simulink model "power_switching"  (Simulink 6.0)
settings: Solver=ode15s  SolverMode=SingleTasking  StartTime=0.0  StopTime=.2  RelTol=1e-4
libraries: powerlib x12, powerlib_extras x1
settings Model: Creator=patrice  LastModifiedBy=batserve  ExtModeTrigMode=oneshot  ExtModeArmWhenConnect=off  ExtModeAutoUpdateStatusClock=off
settings DataIOCC: LimitDataPoints=off  SignalLoggingName=sigsOut
settings OptimizationCC: BlockReduction=off  BooleanDataType=off
settings DebuggingCC: CheckExecutionContextPreStartOutputMsg=on  CheckExecutionContextRuntimeOutputMsg=on  SolverPrmCheckMsg=none  UnconnectedInputMsg=none  UnconnectedOutputMsg=none
settings HardwareCC: TargetUnknown=on
settings RTWCC: TemplateMakefile=grt_vc.tmf

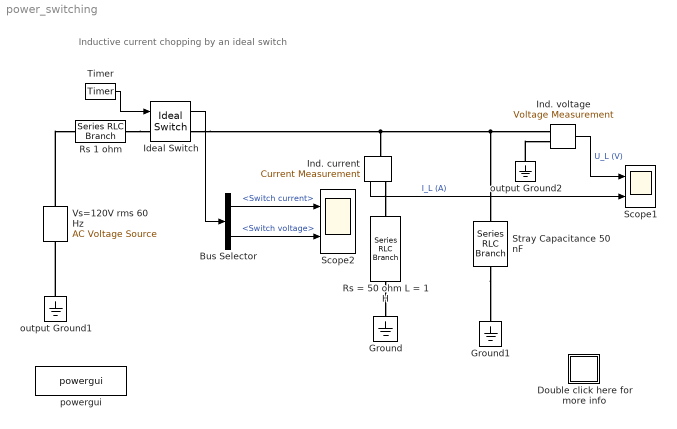
== system power_switching ==
  note: Inductive current chopping by an ideal switch
  "  Ind. current" : powerlib/Measurements/Current Measurement  Tag=PoWeRsYsTeMmEaSuReMeNt  Orientation=down  PhasorSimulation=off  OutputType=Magnitude  PSBequivalent=0
  Bus Selector : BusSelector  DialogController=Simulink.DDGSource_Bus  OutputSignals=Switch current,Switch voltage
  Double click here for more info : Subsystem
      mask Display: disp('?')
  Ground : powerlib/Elements/Ground  Orientation=down  PhysicalDomain=powersysdomain  SubClassName=unknown  LeftPortType=p1  RightPortType=p1  LConnTagsString=a
  Ground1 : powerlib/Elements/Ground  Orientation=down  PhysicalDomain=powersysdomain  SubClassName=unknown  LeftPortType=p1  RightPortType=p1  LConnTagsString=a
  Ideal Switch : powerlib/Power Electronics/Ideal Switch  Ron=1e-3  Lon=1e-9  IC=1  Rs=Inf  Cs=0  Measurements=on
      settings: AttributesFormatString=\n
  Ind. voltage : powerlib/Measurements/Voltage Measurement  Tag=PoWeRsYsTeMmEaSuReMeNt  PhasorSimulation=off  OutputType=Magnitude  PSBequivalent=0
  Rs 1 ohm : powerlib/Elements/Series RLC Branch  PhysicalDomain=powersysdomain  SubClassName=unknown  LeftPortType=p1  RightPortType=p1  LConnTagsString=__new0  RConnTagsString=__new0  Resistance=1  Inductance=0  Capacitance=Inf  Measurements=None
  Rs = 50 ohm L = 1 H : powerlib/Elements/Series RLC Branch  Orientation=down  PhysicalDomain=powersysdomain  SubClassName=unknown  LeftPortType=p1  RightPortType=p1  LConnTagsString=__new0  RConnTagsString=__new0  Resistance=50  Inductance=1  Capacitance=Inf  Measurements=None
  Scope1 : Scope  NumInputPorts=2
      settings: TimeRange=0.2  YMin=-1000~-0.477505  YMax=1000~0.928922  SaveName=U_L  DataFormat=Array
  Scope2 : Scope  NumInputPorts=2
      settings: TimeRange=0.2  YMin=-30~-1000  YMax=10~1000  DataFormat=Array
  Stray Capacitance 50 nF : powerlib/Elements/Series RLC Branch  Orientation=down  PhysicalDomain=powersysdomain  SubClassName=unknown  LeftPortType=p1  RightPortType=p1  LConnTagsString=__new0  RConnTagsString=__new0  Resistance=0  Inductance=0  Capacitance=50e-9  Measurements=None
  Timer : powerlib_extras/Control  Blocks/Timer  t=[0 36e-3 150e-3]  e=[1 0 1 ]
  Vs=120V rms 60 Hz : powerlib/Electrical Sources/AC Voltage Source  Description=source block  Orientation=up  Amplitude=120*sqrt(2)  Phase=0  Frequency=60  SampleTime=0  Measurements=None
      settings: AttributesFormatString=\n
  output Ground1 : powerlib/Elements/Ground  Orientation=down  PhysicalDomain=powersysdomain  SubClassName=unknown  LeftPortType=p1  RightPortType=p1  LConnTagsString=a
  output Ground2 : powerlib/Elements/Ground  Orientation=down  PhysicalDomain=powersysdomain  SubClassName=unknown  LeftPortType=p1  RightPortType=p1  LConnTagsString=a
  powergui : powerlib/powergui  Priority=2  Frange=logspace(0,3,50)  Ylog=off  Xlog=off  save=off  variable=ZData  ZoomFFT=on  StartTime=0.0  cycles=1  DisplayStyle=off  fundamental=60  FreqAxis=off  MaxFrequency=1000  frequencyindice=1  frequencyindicesteady=1  RmsSteady=1  display=off  Ts=0  methode=off  frequency=60  echomessages=on
  wires:
  Bus Selector/1 -> Scope2/1  "<Switch current>"
  Bus Selector/2 -> Scope2/2  "<Switch voltage>"
  Ind. voltage/1 -> Scope1/1  "U_L (V)"
  Timer/1 -> Ideal Switch/1
  Ideal Switch/1 -> Bus Selector/1
  "  Ind. current"/1 -> Scope1/2  "I_L (A)"
  connections:
  Rs 1 ohm/RConn1 -- Ideal Switch/LConn1
  Vs=120V rms 60 Hz/RConn1 -- Rs 1 ohm/LConn1
  output Ground1/LConn1 -- Vs=120V rms 60 Hz/LConn1
  "  Ind. current"/RConn1 -- Rs = 50 ohm L = 1 H/LConn1
  Stray Capacitance 50 nF/RConn1 -- Ground1/LConn1
  output Ground2/LConn1 -- Ind. voltage/LConn2
  Rs = 50 ohm L = 1 H/RConn1 -- Ground/LConn1
  Ideal Switch/RConn1 -- "  Ind. current"/LConn1 -- Ind. voltage/LConn1 -- Stray Capacitance 50 nF/LConn1

== system power_switching/Double click here for more info ==
  note: This example illustrates the effect of current chopping in an inductive circuit
  note: Circuit Description
  note: The  Ideal Switch is used to switch off and on an  inductor (L = 1H, R = 50 ohms) on a 120 Vrms,  60 Hz source.
      | The inductor has a stray capacitance C = 50 nF. The switch resistance  is 1e-3 ohm.
      | The switch is initially closed (initial state = 1). It is open at time t = 36ms and then reclosed at time t = 0.15 s.
  note: Demonstration
  note: G. Sybille (Hydro-Quebec)
  note: Start the simulation.and observe the inductor voltage U_L and inductor  current I_L  on Scope1
      | At the opening time, t = 36 ms, the current in the inductor is I_L= 0.187 A. The current chopping  in the inductor produces a
      | high  frequency overvoltage (711 Hz) across the inductor. The maximum voltage can be calculated from the following equation:
      |
      |      U_Lmax = I_L*sqrt(L/C) = 0.187*sqrt(1/50e-9) = 836 V
      |
      | At the reclosing time, t = 0.15 s, the source voltage is zero. Therefore, a full offset is observed in the inductor current.
      | The switch current spike observed on trace 1 of Scope2 at switch reclosing (t = 0.15 s) is due to the capacitor discharge through
      | the source resistance. If you zoom on this current spike you will observe a current step of 30 A
      | (30V capacitor voltage / 1 ohm source resistance), followed by a fast discharge time constant (RC = 1*50e-9 = 50e-9 s).
